simulink model "f14_digital"  (Simulink 6.0)
settings: Solver=ode45  SolverMode=SingleTasking  StartTime=0.0  StopTime=60  FixedStep=.01  RelTol=1e-4  AbsTol=1e-6
PreLoadFcn:
  | f14dat_digital
values from neighbouring files (symbols this model uses):
  a = 2.5348    [f14dat.m]    (also in f14dat_digital.m; f14def.m)
  b = find_system('aero_atc','Type','block')    [aero_atcscript.m]    (also in f14dat.m = 64.13; f14dat_digital.m = 64.13; f14def.m = 64.13)
  deltat = pinput(23)    [aero_extkalman.m]    (also in aero_raddat.m = 1; f14dat_digital.m = 0.1)
  deltat1 = 0.01    [f14dat_digital.m]
  g = 9.81    [aero_guid_dat.m]    (also in aero_raddat.m = 32.2; f14dat.m = 32.2; f14dat_digital.m = 32.2)
  Ka = 0.6770    (= 0.677)    [f14dat.m]    (also in f14dat_digital.m; f14def.m)
  Kf = -1.7460    (= -1.746)    [f14dat.m]    (also in f14dat_digital.m; f14def.m)
  Ki = -3.8640    (= -3.864)    [f14dat.m]    (also in f14dat_digital.m; f14def.m)
  Kq = 0.8156    [f14dat.m]    (also in f14dat_digital.m; f14def.m)
  Md = -6.8847    [f14dat.m]    (also in f14dat_digital.m; f14def.m)
  Mq = -0.6571    [f14dat.m]    (also in f14dat_digital.m; f14def.m)
  Mw = -0.00592    [f14dat.m]    (also in f14dat_digital.m; f14def.m)
  Swg = 3    [f14dat.m]    (also in f14dat_digital.m; f14def.m)
  Tal = 0.3959    [f14dat.m]    (also in f14dat_digital.m; f14def.m)
  Ts = 0.1000    (= 0.1)    [f14dat.m]    (also in f14dat_digital.m; f14def.m)
  Uo = 689.4000    (= 689.4)    [f14dat.m]    (also in f14dat_digital.m; f14def.m)
  Vto = 690.4000    (= 690.4)    [f14dat.m]    (also in f14dat_digital.m; f14def.m)
  W1 = 2.9710    (= 2.971)    [f14dat.m]    (also in f14dat_digital.m; f14def.m)
  W2 = 4.1440    (= 4.144)    [f14dat.m]    (also in f14dat_digital.m; f14def.m)
  Zd = -63.9979    [f14dat.m]    (also in f14dat_digital.m; f14def.m)
  Zw = -0.6385    [f14dat.m]    (also in f14dat_digital.m; f14def.m)
undefined symbols (not defined in the file or in its folder): DiscIntNeverNeededParam
libraries: simulink x3, f14actuator x1, cstblocks x1
Description:
  | This model of the F14 is used to design a high angle of attack Digital Flight Control System.  The design works in conjunction with the GUI in F14guid.  There is documentation that goes along with this file and the
  | GUI.  The documentaiton is in the Word file "F14 Design.doc".
settings Model: Creator=The MathWorks Inc.  LastModifiedBy=batserve  ExtModeTrigMode=oneshot  ExtModeArmWhenConnect=off  ExtModeAutoUpdateStatusClock=off
settings DataIOCC: ExternalInput=[]  InitialState=[]  LimitDataPoints=off  SaveOutput=off  SaveTime=off  SignalLoggingName=logsOut
settings OptimizationCC: BlockReduction=off  BooleanDataType=off
settings DebuggingCC: CheckExecutionContextPreStartOutputMsg=on  CheckExecutionContextRuntimeOutputMsg=on  SolverPrmCheckMsg=none  IntegerOverflowMsg=none
settings HardwareCC: TargetUnknown=on
settings RTWCC: GenCodeOnly=on  TemplateMakefile=grt_vc.tmf

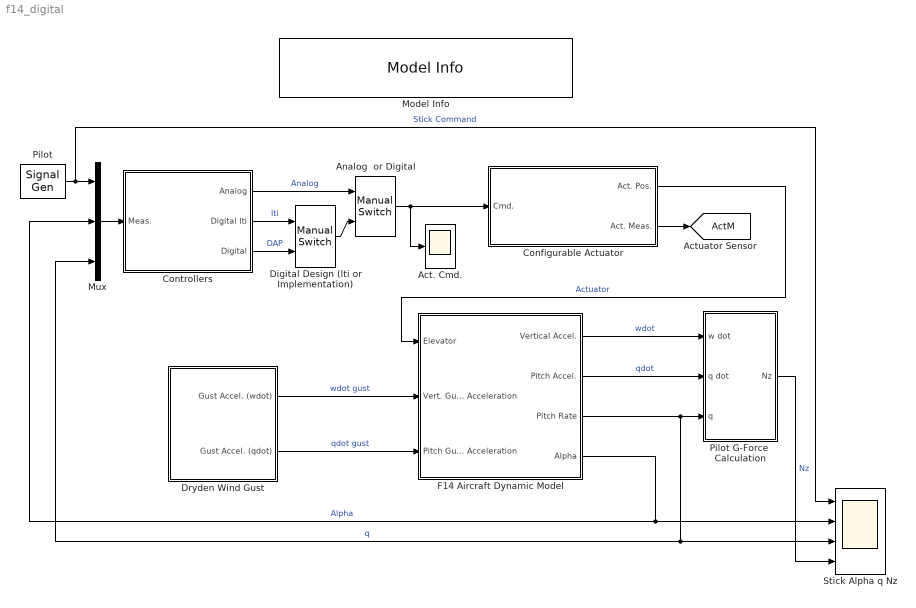
== system f14_digital ==
  Act. Cmd. : Scope
      settings: TickLabels=on  TimeRange=15  YMin=-2.5  YMax=2.5  DataFormat=Array
  Analog  or Digital : simulink/Signal Routing/Manual Switch  sw=1  action=0
  Configurable Actuator : Subsystem  BlockChoice=Linear Actuator Subsystem  PropExecContextAcrossSSBoundary=on
      settings: MemberBlocks=Linear Actuator Subsystem,Non-Linear Actuator Subsystem
      settings: TemplateBlock=|
      | f14actuator/Configurable
      | Actuator
  Controllers : Subsystem  PropExecContextAcrossSSBoundary=on
      mask Display: image(contrgb)
  Digital Design (lti or Implementation) : simulink/Signal Routing/Manual Switch  sw=1  action=0
  Dryden Wind Gust : Subsystem  PropExecContextAcrossSSBoundary=on
      mask Display: image(weatherrgb)
  F14 Aircraft Dynamic Model : Subsystem  PropExecContextAcrossSSBoundary=on
      mask Display: image(rgb)
  Model Info : simulink/Model-Wide Utilities/Model Info  InitialBlockCM=none  BlockCM=none  Frame=off  DisplayStringWithTags="F14 High Angle of Attack  Digital Flight Control System"  HorizontalTextAlignment=Center  LeftAlignmentValue=0.5  SourceBlockDiagram=f14_digital  TagMaxNumber=20
  Mux : Mux  Inputs=3
  Pilot : SignalGenerator  WaveForm=square  Frequency=.1
  Pilot G-Force  Calculation : Subsystem  PropExecContextAcrossSSBoundary=on
  Stick Alpha q Nz : Scope  NumInputPorts=4
      settings: TickLabels=on  TimeRange=15  YMin=-1~-1.5~-3~-15  YMax=1~1.5~3~15  DataFormat=Array
  tag scope: ActM=global
  wires:
  Controllers/3(Digital) -> Digital Design (lti or Implementation)/2  "DAP"
  Controllers/2(Digital lti) -> Digital Design (lti or Implementation)/1  "lti"
  Digital Design (lti or Implementation)/1 -> Analog  or Digital/2
  Configurable Actuator/1(Act. Pos.) -> F14 Aircraft Dynamic Model/1(Elevator)  "Actuator"
  Controllers/1(Analog) -> Analog  or Digital/1  "Analog"
  Mux/1 -> Controllers/1(Meas.)
  F14 Aircraft Dynamic Model/1(Vertical Accel.) -> Pilot G-Force  Calculation/1(w dot)  "wdot"
  F14 Aircraft Dynamic Model/2(Pitch Accel.) -> Pilot G-Force  Calculation/2(q dot)  "qdot"
  Pilot/1 -> Mux/1, Stick Alpha q Nz/1  "Stick Command"
  F14 Aircraft Dynamic Model/4(Alpha) -> Mux/2, Stick Alpha q Nz/2  "Alpha"
  Configurable Actuator/2(Act. Meas.) -> [ActM]
  Dryden Wind Gust/2(Gust Accel. (qdot)) -> F14 Aircraft Dynamic Model/3(Pitch Gust Acceleration)  "qdot gust"
  Dryden Wind Gust/1(Gust Accel. (wdot)) -> F14 Aircraft Dynamic Model/2(Vert. Gust Acceleration)  "wdot gust"
  F14 Aircraft Dynamic Model/3(Pitch Rate) -> Pilot G-Force  Calculation/3(q), Stick Alpha q Nz/3, Mux/3  "q"
  Pilot G-Force  Calculation/1(Nz) -> Stick Alpha q Nz/4  "Nz"
  Analog  or Digital/1 -> Configurable Actuator/1(Cmd.), Act. Cmd./1

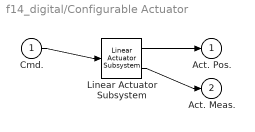
== system f14_digital/Configurable Actuator ==
  Cmd. : Inport  Port=1  LatchInput=off
  Linear Actuator Subsystem : f14actuator/Linear Actuator Subsystem
  Act. Pos. : Outport
  Act. Meas. : Outport  Port=2
  wires:
  Cmd./1 -> Linear Actuator Subsystem/1
  Linear Actuator Subsystem/1 -> Act. Pos./1
  Linear Actuator Subsystem/2 -> Act. Meas./1

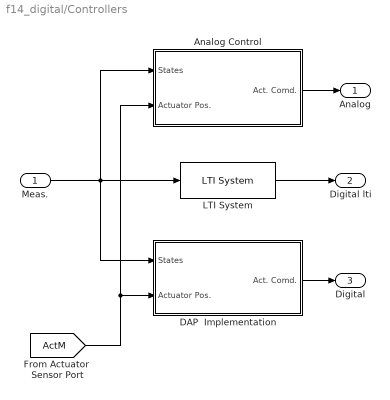
== system f14_digital/Controllers ==
  Meas. : Inport  Port=1  LatchInput=off
  Analog Control : Subsystem  PropExecContextAcrossSSBoundary=on
  DAP  Implementation : Subsystem  PropExecContextAcrossSSBoundary=on
  LTI System : cstblocks/LTI System  sys=discap  IC=[0]
  Analog : Outport
  Digital lti : Outport  Port=2
  Digital : Outport  Port=3
  wires:
  Meas./1 -> LTI System/1, DAP  Implementation/1(States), Analog Control/1(States)
  [ActM] -> DAP  Implementation/2(Actuator Pos.), Analog Control/2(Actuator Pos.)
  LTI System/1 -> Digital lti/1
  DAP  Implementation/1(Act. Comd.) -> Digital/1
  Analog Control/1(Act. Comd.) -> Analog/1

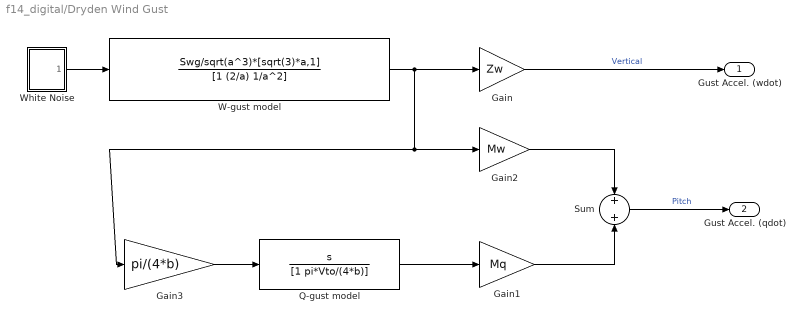
== system f14_digital/Dryden Wind Gust ==
  Gain : Gain  Gain=Zw  SaturateOnIntegerOverflow=on
  Gain1 : Gain  Gain=Mq  SaturateOnIntegerOverflow=on
  Gain2 : Gain  Gain=Mw  SaturateOnIntegerOverflow=on
  Gain3 : Gain  Gain=pi/(4*b)  SaturateOnIntegerOverflow=on
  Q-gust model : TransferFcn  Numerator=[1 0]  Denominator=[1 pi*Vto/(4*b)]
  Sum : Sum  SaturateOnIntegerOverflow=on  InputSameDT=on
  W-gust model : TransferFcn  Numerator=Swg/sqrt(a^3)*[sqrt(3)*a,1]  Denominator=[1 (2/a) 1/a^2]
  White Noise : Subsystem  PropExecContextAcrossSSBoundary=on  mask(Continuous White Noise.){Cov=10, Ts=0.01, seed=23341}
      mask prompts: Cov "Noise Variance:"; Ts "Sample Time:"
      mask help:
      | White noise for continuous (s-domain) systems.
      | Band-limited using zero-order-hold.
      mask init:
      | r = rand(1,12); r2 = [r(1),r;r,r(12)]; t =[1:13;1:13];
      mask Help: Implemented using white noise into Zero Order Hold block. For faster simulation set sample time to highest value possible but in accordance with the fastest dynamics of system.
      mask Display: plot(t(:),r2(:))
  Gust Accel. (wdot) : Outport
  Gust Accel. (qdot) : Outport  Port=2
  wires:
  Gain/1 -> Gust Accel. (wdot)/1  "Vertical"
  White Noise/1(out_1) -> W-gust model/1
  Gain3/1 -> Q-gust model/1
  Sum/1 -> Gust Accel. (qdot)/1  "Pitch"
  Gain2/1 -> Sum/1
  Gain1/1 -> Sum/2
  Q-gust model/1 -> Gain1/1
  W-gust model/1 -> Gain/1, Gain2/1, Gain3/1

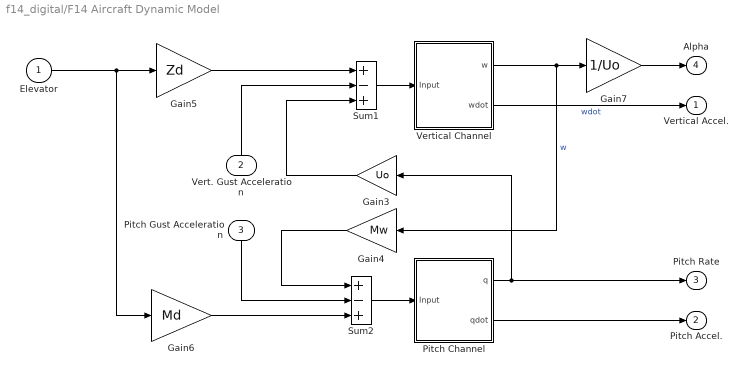
== system f14_digital/F14 Aircraft Dynamic Model ==
  Elevator : Inport  Port=1  LatchInput=off
  Vert. Gust Acceleration : Inport  Orientation=up  Port=2  LatchInput=off
  Pitch Gust Acceleration : Inport  Orientation=down  Port=3  LatchInput=off
  Gain3 : Gain  Orientation=left  Gain=Uo  SaturateOnIntegerOverflow=on
  Gain4 : Gain  Orientation=left  Gain=Mw  SaturateOnIntegerOverflow=on
  Gain5 : Gain  Gain=Zd  SaturateOnIntegerOverflow=on
  Gain6 : Gain  Gain=Md  SaturateOnIntegerOverflow=on
  Gain7 : Gain  Gain=1/Uo  SaturateOnIntegerOverflow=on
  Pitch Channel : Subsystem  PropExecContextAcrossSSBoundary=on
  Sum1 : Sum  Inputs=+-+  SaturateOnIntegerOverflow=on  InputSameDT=on
  Sum2 : Sum  Inputs=+-+  SaturateOnIntegerOverflow=on  InputSameDT=on
  Vertical Channel : Subsystem  PropExecContextAcrossSSBoundary=on
  Vertical Accel. : Outport  InitialOutput=0
  Pitch Accel. : Outport  Port=2  InitialOutput=0
  Pitch Rate : Outport  Port=3  InitialOutput=0
  Alpha : Outport  Port=4  InitialOutput=0
  wires:
  Pitch Channel/2(qdot) -> Pitch Accel./1
  Pitch Channel/1(q) -> Pitch Rate/1, Gain3/1
  Vertical Channel/2(wdot) -> Vertical Accel./1  "wdot"
  Vertical Channel/1(w) -> Gain4/1, Gain7/1  "w"
  Sum1/1 -> Vertical Channel/1(Input)
  Gain6/1 -> Sum2/3
  Gain5/1 -> Sum1/1
  Pitch Gust Acceleration/1 -> Sum2/2
  Sum2/1 -> Pitch Channel/1(Input)
  Vert. Gust Acceleration/1 -> Sum1/2
  Elevator/1 -> Gain5/1, Gain6/1
  Gain7/1 -> Alpha/1
  Gain3/1 -> Sum1/3
  Gain4/1 -> Sum2/1

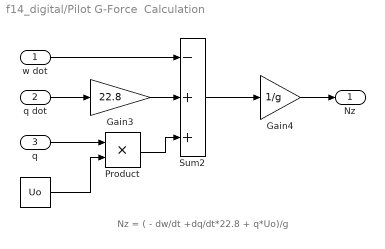
== system f14_digital/Pilot G-Force  Calculation ==
  note: Nz = ( - dw/dt +dq/dt*22.8 + q*Uo)/g
  w dot : Inport  Port=1  LatchInput=off
  q dot : Inport  Port=2  LatchInput=off
  q : Inport  Port=3  LatchInput=off
  " " : Constant  Value=Uo
  Gain3 : Gain  Gain=22.8  SaturateOnIntegerOverflow=on
  Gain4 : Gain  Gain=1/g  SaturateOnIntegerOverflow=on
  Product : Product  SaturateOnIntegerOverflow=on  RndMeth=Zero  InputSameDT=on
  Sum2 : Sum  Inputs=-++  SaturateOnIntegerOverflow=on  InputSameDT=on
  Nz : Outport  InitialOutput=0
  wires:
  Sum2/1 -> Gain4/1
  w dot/1 -> Sum2/1
  Gain4/1 -> Nz/1
  q dot/1 -> Gain3/1
  Gain3/1 -> Sum2/2
  Product/1 -> Sum2/3
  q/1 -> Product/1
  " "/1 -> Product/2

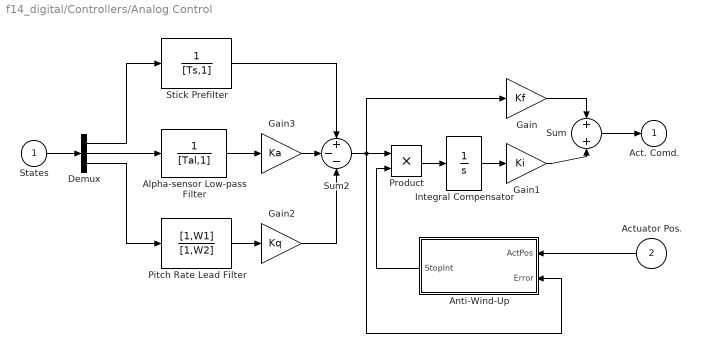
== system f14_digital/Controllers/Analog Control ==
  States : Inport  Port=1  LatchInput=off
  Actuator Pos. : Inport  Orientation=left  Port=2  LatchInput=off
  Alpha-sensor Low-pass Filter : TransferFcn  Denominator=[Tal,1]
  Anti-Wind-Up : Stateflow chart  Orientation=left  PropExecContextAcrossSSBoundary=on
  Demux : Demux  Outputs=3
  Gain : Gain  Gain=Kf  SaturateOnIntegerOverflow=on
  Gain1 : Gain  Gain=Ki  SaturateOnIntegerOverflow=on
  Gain2 : Gain  Gain=Kq  SaturateOnIntegerOverflow=on
  Gain3 : Gain  Gain=Ka  SaturateOnIntegerOverflow=on
  Integral Compensator : TransferFcn  Denominator=[1,0]
  Pitch Rate Lead Filter : TransferFcn  Numerator=[1,W1]  Denominator=[1,W2]
  Product : Product  SaturateOnIntegerOverflow=on  RndMeth=Zero  InputSameDT=on
  Stick Prefilter : TransferFcn  Denominator=[Ts,1]
  Sum : Sum  Inputs=2  SaturateOnIntegerOverflow=on  InputSameDT=on
  Sum2 : Sum  Inputs=+--  SaturateOnIntegerOverflow=on  InputSameDT=on
  Act. Comd. : Outport  InitialOutput=0
  wires:
  Actuator Pos./1 -> Anti-Wind-Up/1(ActPos)
  Anti-Wind-Up/1(StopInt) -> Product/2
  Sum2/1 -> Anti-Wind-Up/2(Error), Gain/1, Product/1
  Product/1 -> Integral Compensator/1
  Integral Compensator/1 -> Gain1/1
  Sum/1 -> Act. Comd./1
  States/1 -> Demux/1
  Alpha-sensor Low-pass Filter/1 -> Gain3/1
  Gain2/1 -> Sum2/3
  Stick Prefilter/1 -> Sum2/1
  Pitch Rate Lead Filter/1 -> Gain2/1
  Demux/1 -> Stick Prefilter/1
  Demux/2 -> Alpha-sensor Low-pass Filter/1
  Demux/3 -> Pitch Rate Lead Filter/1
  Gain3/1 -> Sum2/2
  Gain/1 -> Sum/1
  Gain1/1 -> Sum/2

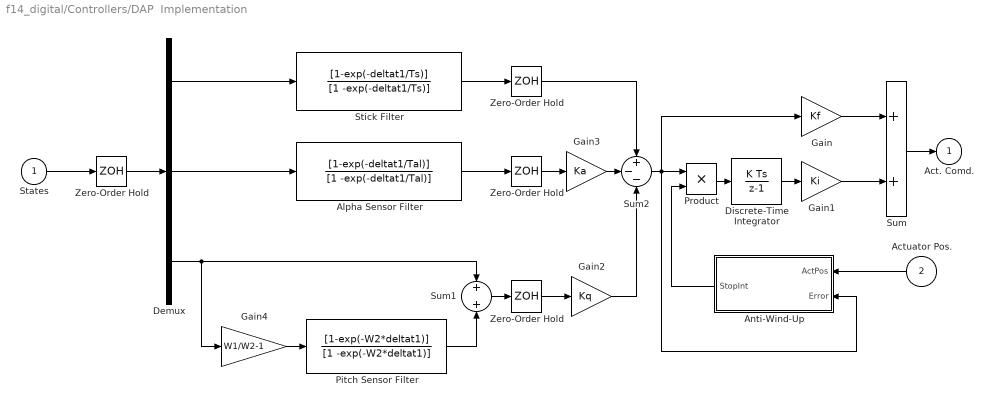
== system f14_digital/Controllers/DAP  Implementation ==
  States : Inport  Port=1  LatchInput=off
  Actuator Pos. : Inport  Orientation=left  Port=2  LatchInput=off
  Alpha Sensor Filter : DiscreteTransferFcn  Numerator=[1-exp(-deltat1/Tal)]  Denominator=[1 -exp(-deltat1/Tal)]  SampleTime=deltat1
  Anti-Wind-Up : Stateflow chart  Orientation=left  PropExecContextAcrossSSBoundary=on
  Demux : Demux  Outputs=3
  Discrete-Time Integrator : DiscreteIntegrator  SampleTime=deltat  ICPrevOutput=DiscIntNeverNeededParam  ICPrevScaledInput=DiscIntNeverNeededParam
  Gain : Gain  Gain=Kf  SaturateOnIntegerOverflow=on
  Gain1 : Gain  Gain=Ki  SaturateOnIntegerOverflow=on
  Gain2 : Gain  Gain=Kq  SaturateOnIntegerOverflow=on
  Gain3 : Gain  Gain=Ka  SaturateOnIntegerOverflow=on
  Gain4 : Gain  Gain=W1/W2-1  SaturateOnIntegerOverflow=on
  Pitch Sensor Filter : DiscreteTransferFcn  Numerator=[1-exp(-W2*deltat1)]  Denominator=[1 -exp(-W2*deltat1)]  SampleTime=deltat1
  Product : Product  SaturateOnIntegerOverflow=on  RndMeth=Zero  InputSameDT=on
  Stick Filter : DiscreteTransferFcn  Numerator=[1-exp(-deltat1/Ts)]  Denominator=[1 -exp(-deltat1/Ts)]  SampleTime=deltat1
  Sum : Sum  Inputs=2  SaturateOnIntegerOverflow=on  InputSameDT=on
  Sum1 : Sum  Inputs=2  SaturateOnIntegerOverflow=on  InputSameDT=on
  Sum2 : Sum  Inputs=+--  SaturateOnIntegerOverflow=on  InputSameDT=on
  Zero-Order Hold : ZeroOrderHold  SampleTime=deltat
  "Zero-Order Hold " : ZeroOrderHold  SampleTime=deltat1
  "Zero-Order Hold  " : ZeroOrderHold  SampleTime=deltat
  "Zero-Order Hold   " : ZeroOrderHold  SampleTime=deltat
  Act. Comd. : Outport  InitialOutput=0
  wires:
  Sum/1 -> Act. Comd./1
  Discrete-Time Integrator/1 -> Gain1/1
  Product/1 -> Discrete-Time Integrator/1
  Sum2/1 -> Product/1, Gain/1, Anti-Wind-Up/2(Error)
  Anti-Wind-Up/1(StopInt) -> Product/2
  Actuator Pos./1 -> Anti-Wind-Up/1(ActPos)
  Demux/2 -> Alpha Sensor Filter/1
  Demux/1 -> Stick Filter/1
  Stick Filter/1 -> Zero-Order Hold/1
  Zero-Order Hold/1 -> Sum2/1
  Alpha Sensor Filter/1 -> "Zero-Order Hold  "/1
  "Zero-Order Hold  "/1 -> Gain3/1
  States/1 -> "Zero-Order Hold "/1
  "Zero-Order Hold "/1 -> Demux/1
  Gain3/1 -> Sum2/2
  Gain/1 -> Sum/1
  Gain1/1 -> Sum/2
  Gain2/1 -> Sum2/3
  Demux/3 -> Sum1/1, Gain4/1
  Sum1/1 -> "Zero-Order Hold   "/1
  Pitch Sensor Filter/1 -> Sum1/2
  Gain4/1 -> Pitch Sensor Filter/1
  "Zero-Order Hold   "/1 -> Gain2/1

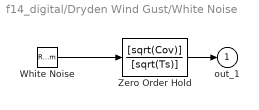
== system f14_digital/Dryden Wind Gust/White Noise ==
  White Noise : RandomNumber  Seed=seed  SampleTime=Ts
  Zero Order Hold : DiscreteTransferFcn  Numerator=[sqrt(Cov)]  Denominator=[sqrt(Ts)]  SampleTime=Ts
  out_1 : Outport  InitialOutput=0
  wires:
  Zero Order Hold/1 -> out_1/1
  White Noise/1 -> Zero Order Hold/1

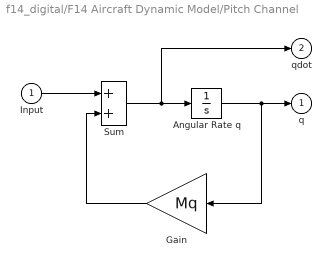
== system f14_digital/F14 Aircraft Dynamic Model/Pitch Channel ==
  Input : Inport  Port=1  LatchInput=off
  "Angular Rate q " : Integrator
  Gain : Gain  Orientation=left  Gain=Mq  SaturateOnIntegerOverflow=on
  Sum : Sum  SaturateOnIntegerOverflow=on  InputSameDT=on
  q : Outport  InitialOutput=0
  qdot : Outport  Port=2  InitialOutput=0
  wires:
  Input/1 -> Sum/1
  Gain/1 -> Sum/2
  "Angular Rate q "/1 -> q/1, Gain/1
  Sum/1 -> "Angular Rate q "/1, qdot/1

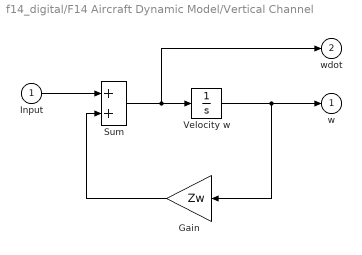
== system f14_digital/F14 Aircraft Dynamic Model/Vertical Channel ==
  Input : Inport  Port=1  LatchInput=off
  Gain : Gain  Orientation=left  Gain=Zw  SaturateOnIntegerOverflow=on
  Sum : Sum  SaturateOnIntegerOverflow=on  InputSameDT=on
  Velocity w : Integrator
  w : Outport  InitialOutput=0
  wdot : Outport  Port=2  InitialOutput=0
  wires:
  Sum/1 -> wdot/1, Velocity w/1
  Velocity w/1 -> Gain/1, w/1
  Gain/1 -> Sum/2
  Input/1 -> Sum/1

== stateflow chart Controllers/DAP Implementation/Anti-Wind-Up ==
  state Integrate
    en:StopInt=1;
  state Stop_Integrating
    en: StopInt=0;
  (default) -> Integrate
  Integrate -> Stop_Integrating : [(ActPos>Sat & Error > 0) | (ActPos<-Sat & Error < 0) ]
  Stop_Integrating -> Integrate : [ActPos<Sat & ActPos>-Sat ]
  data: ActPos input double; Error input double; StopInt output double; Sat constant double =0.785398

== stateflow chart Controllers/Analog Control/Anti-Wind-Up ==
  state Integrate
    en:StopInt=1;
  state Stop_Integrating
    en: StopInt=0;
  (default) -> Integrate
  Integrate -> Stop_Integrating : [(ActPos>Sat & Error > 0) | (ActPos<-Sat & Error < 0) ]
  Stop_Integrating -> Integrate : [ActPos<Sat & ActPos>-Sat]
  data: ActPos input double; Error input double; StopInt output double; Sat constant double =0.785398
